simulink model "smallsat_adcs"  (R2025b)
settings: Solver=ode113  StartTime=0.0  StopTime=17403  RelTol=1e-10  AbsTol=1e-10
InitFcn:
  | P = smallsat_params; if ~exist('adcsCase', 'var'), adcsCase = 'tumble'; end; ic = initial_state_case(P, adcsCase); bdot = size_bdot(P); pointing = size_pointing(P);
undefined symbols (not defined in the file or in its folder): DiscIntNeverNeededParam, magnetic_field_eci, quat_to_dcm
libraries: aerolibutil x3, matrix_library x1, simulink x1, sharedutil x1
settings Model: Creator=USER  LastModifiedBy=USER

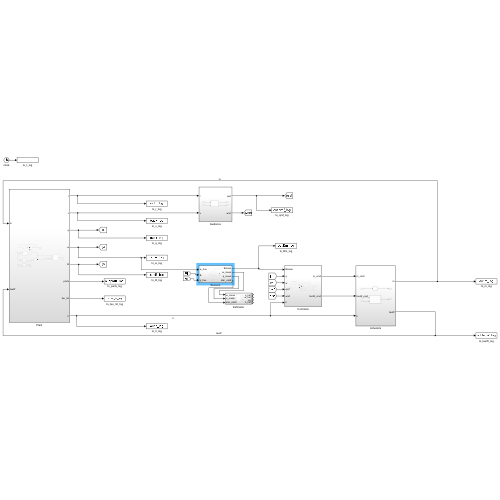
[thumbnail: Simulink's stored preview of the top-level diagram]
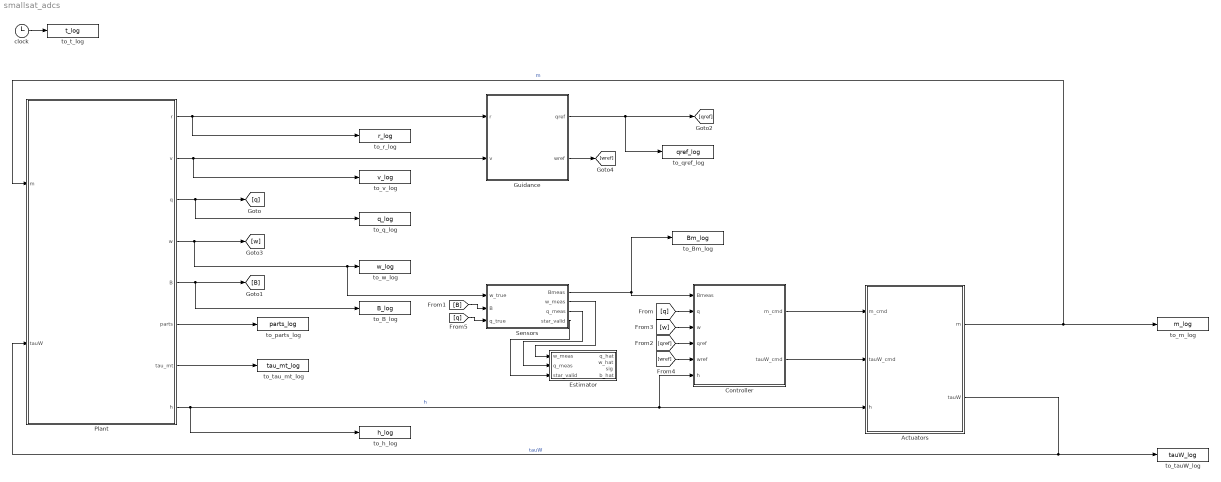
== system smallsat_adcs ==
  Actuators : Subsystem
  Controller : Subsystem
  Estimator : Subsystem
  Guidance : Subsystem
  Plant : Subsystem
  Sensors : Subsystem
  clock : Clock
  to_B_log : ToWorkspace  VariableName=B_log  SampleTime=10
  to_Bm_log : ToWorkspace  VariableName=Bm_log  SampleTime=10
  to_h_log : ToWorkspace  VariableName=h_log  SampleTime=10
  to_m_log : ToWorkspace  VariableName=m_log  SampleTime=10
  to_parts_log : ToWorkspace  VariableName=parts_log  SampleTime=10
  to_q_log : ToWorkspace  VariableName=q_log  SampleTime=10
  to_qref_log : ToWorkspace  VariableName=qref_log  SampleTime=10
  to_r_log : ToWorkspace  VariableName=r_log  SampleTime=10
  to_t_log : ToWorkspace  VariableName=t_log  SampleTime=10
  to_tauW_log : ToWorkspace  VariableName=tauW_log  SampleTime=10
  to_tau_mt_log : ToWorkspace  VariableName=tau_mt_log  SampleTime=10
  to_v_log : ToWorkspace  VariableName=v_log  SampleTime=10
  to_w_log : ToWorkspace  VariableName=w_log  SampleTime=10
  wires:
  Plant/5(B) -> to_B_log/1, [B]
  Plant/1(r) -> Guidance/1(r), to_r_log/1
  Plant/2(v) -> to_v_log/1, Guidance/2(v)
  Sensors/1(Bmeas) -> Controller/1(Bmeas), to_Bm_log/1
  Plant/3(q) -> to_q_log/1, [q]
  Guidance/1(qref) -> to_qref_log/1, [qref]
  Controller/1(m_cmd) -> Actuators/1(m_cmd)
  Controller/2(tauW_cmd) -> Actuators/2(tauW_cmd)
  Plant/8(h) -> to_h_log/1, Actuators/3(h), Controller/6(h)  "h"
  Actuators/1(m) -> to_m_log/1, Plant/1(m)  "m"
  Actuators/2(tauW) -> to_tauW_log/1, Plant/2(tauW)  "tauW"
  clock/1 -> to_t_log/1
  Plant/6(parts) -> to_parts_log/1
  Plant/7(tau_mt) -> to_tau_mt_log/1
  [q] -> Controller/2(q)
  [B] -> Sensors/2(B)
  [qref] -> Controller/4(qref)
  [w] -> Controller/3(w)
  Guidance/2(wref) -> [wref]
  [wref] -> Controller/5(wref)
  Plant/4(w) -> Sensors/1(w_true), to_w_log/1, [w]
  [q] -> Sensors/3(q_true)
  Sensors/2(w_meas) -> Estimator/1(w_meas)
  Sensors/3(q_meas) -> Estimator/2(q_meas)
  Sensors/4(star_valid) -> Estimator/3(star_valid)

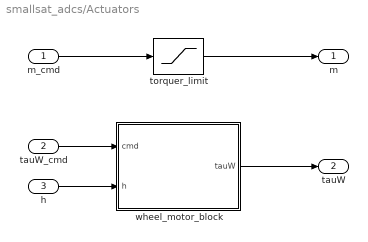
== system smallsat_adcs/Actuators ==
  m_cmd : Inport
  tauW_cmd : Inport  Port=2
  h : Inport  Port=3
  torquer_limit : Saturate  UpperLimit=P.mtqMax  LowerLimit=-P.mtqMax
  wheel_motor_block : MATLAB Function  TreatAsAtomicUnit=on
  m : Outport
  tauW : Outport  Port=2
  wires:
  m_cmd/1 -> torquer_limit/1
  torquer_limit/1 -> m/1
  tauW_cmd/1 -> wheel_motor_block/1(cmd)
  h/1 -> wheel_motor_block/2(h)
  wheel_motor_block/1(tauW) -> tauW/1

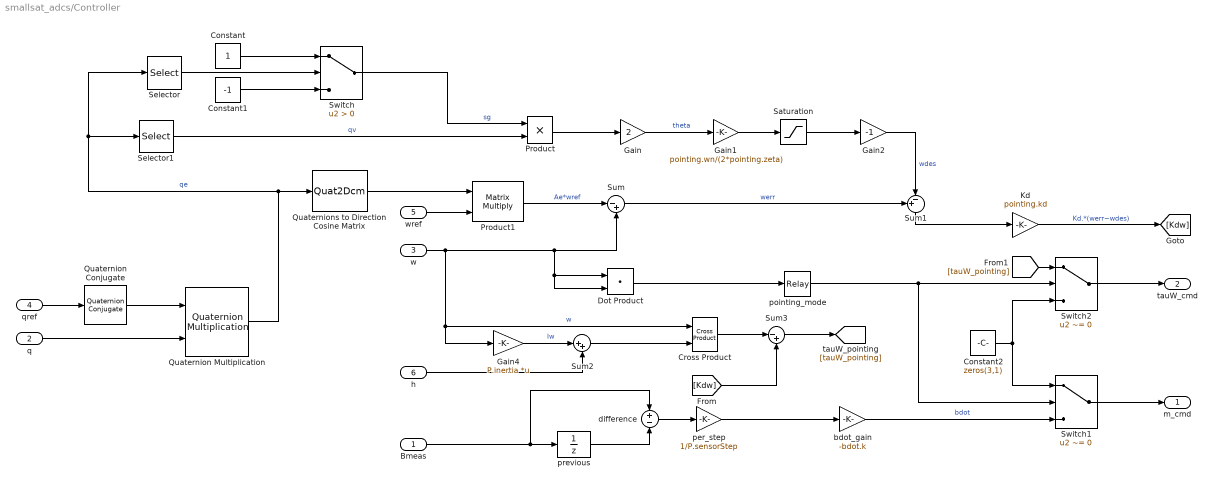
== system smallsat_adcs/Controller ==
  Bmeas : Inport
  q : Inport  Port=2
  w : Inport  Port=3
  qref : Inport  Port=4
  wref : Inport  Port=5
  h : Inport  Port=6
  Constant : Constant
  Constant1 : Constant  Value=-1
  Constant2 : Constant  Value=zeros(3,1)  VectorParams1D=off
  Cross Product : matrix_library/Cross Product
  Dot Product : DotProduct  OutDataTypeStr=Inherit: Inherit via internal rule
  Gain : Gain  Gain=2
  Gain1 : Gain  Gain=pointing.wn/(2*pointing.zeta)
  Gain2 : Gain  Gain=-1
  Gain4 : Gain  Gain=P.inertia  Multiplication=Matrix(K*u)
  Kd : Gain  Gain=pointing.kd
  Product : Product
  Product1 : Product  Multiplication=Matrix(*)
  Quaternion Conjugate : aerolibutil/Quaternion Conjugate
  Quaternion Multiplication : aerolibutil/Quaternion Multiplication
  Quaternions to Direction Cosine Matrix : Quat2Dcm
  Saturation : Saturate  UpperLimit=pointing.wSlew  LowerLimit=-pointing.wSlew
  Selector : Selector  InputPortWidth=4  IndexOptions=Index vector (dialog)  Indices=1  OutputSizes=1
  Selector1 : Selector  InputPortWidth=4  IndexOptions=Index vector (dialog)  Indices=[2 3 4]  OutputSizes=1
  Sum : Sum  Inputs=|-+
  Sum1 : Sum  Inputs=+-|
  Sum2 : Sum  Inputs=|++
  Sum3 : Sum  Inputs=|-+
  Switch : Switch  Criteria=u2 > Threshold  SaturateOnIntegerOverflow=off  InputSameDT=off
  Switch1 : Switch  Criteria=u2 ~= 0  SaturateOnIntegerOverflow=off  InputSameDT=off
  Switch2 : Switch  Criteria=u2 ~= 0  SaturateOnIntegerOverflow=off  InputSameDT=off
  bdot_gain : Gain  Gain=-bdot.k
  difference : Sum  Inputs=+-
  per_step : Gain  Gain=1/P.sensorStep
  pointing_mode : Relay  OnSwitchValue=P.detumbleExit^2  OffSwitchValue=P.detumbleTarget^2  OnOutputValue=0  OffOutputValue=1
  previous : UnitDelay  InitialCondition=quat_to_dcm(ic.q)*magnetic_field_eci(ic.r, 0, P)  SampleTime=P.sensorStep  HasFrameUpgradeWarning=on
  m_cmd : Outport
  tauW_cmd : Outport  Port=2
  wires:
  w/1 -> Cross Product/1, Gain4/1, Sum/2, Dot Product/2, Dot Product/1  "w"
  wref/1 -> Product1/2
  Bmeas/1 -> difference/1, previous/1
  previous/1 -> difference/2
  difference/1 -> per_step/1
  per_step/1 -> bdot_gain/1
  bdot_gain/1 -> Switch1/3  "bdot"
  Switch2/1 -> tauW_cmd/1
  qref/1 -> Quaternion Conjugate/1
  Quaternion Conjugate/1 -> Quaternion Multiplication/1
  q/1 -> Quaternion Multiplication/2
  Quaternion Multiplication/1 -> Quaternions to Direction Cosine Matrix/1, Selector/1, Selector1/1  "qe"
  Constant/1 -> Switch/1
  Selector/1 -> Switch/2
  Constant1/1 -> Switch/3
  Switch/1 -> Product/1  "sg"
  Selector1/1 -> Product/2  "qv"
  Product/1 -> Gain/1
  Gain/1 -> Gain1/1  "theta"
  Gain1/1 -> Saturation/1
  Saturation/1 -> Gain2/1
  Gain2/1 -> Sum1/2  "wdes"
  Quaternions to Direction Cosine Matrix/1 -> Product1/1
  Product1/1 -> Sum/1  "Ae*wref"
  Sum/1 -> Sum1/1  "werr"
  Sum1/1 -> Kd/1
  Kd/1 -> [Kdw]  "Kd.*(werr−wdes)"
  Dot Product/1 -> pointing_mode/1
  Constant2/1 -> Switch2/3, Switch1/1
  pointing_mode/1 -> Switch2/2, Switch1/2
  Switch1/1 -> m_cmd/1
  Gain4/1 -> Sum2/1  "Iw"
  h/1 -> Sum2/2
  Sum2/1 -> Cross Product/2
  Cross Product/1 -> Sum3/1
  [Kdw] -> Sum3/2
  Sum3/1 -> [tauW_pointing]
  [tauW_pointing] -> Switch2/1

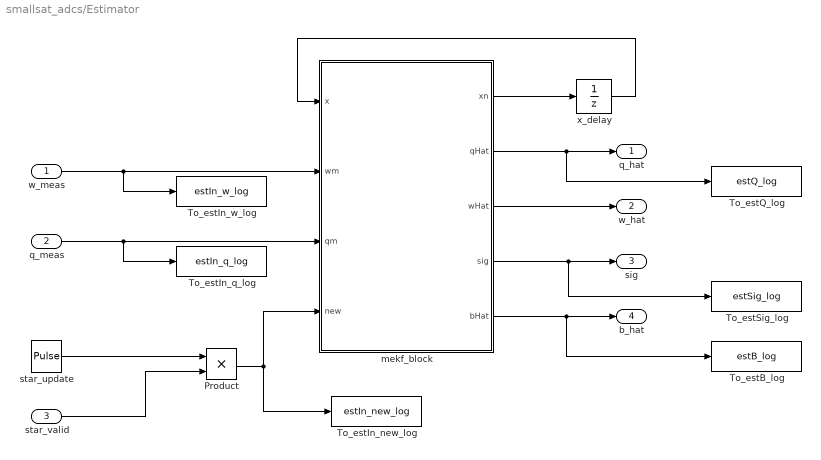
== system smallsat_adcs/Estimator ==
  w_meas : Inport
  q_meas : Inport  Port=2
  star_valid : Inport  Port=3
  Product : Product
  To_estB_log : ToWorkspace  VariableName=estB_log  SampleTime=-1
  To_estIn_new_log : ToWorkspace  VariableName=estIn_new_log  SampleTime=-1
  To_estIn_q_log : ToWorkspace  VariableName=estIn_q_log  SampleTime=P.gyroStep
  To_estIn_w_log : ToWorkspace  VariableName=estIn_w_log  SampleTime=-1
  To_estQ_log : ToWorkspace  VariableName=estQ_log  SampleTime=-1
  To_estSig_log : ToWorkspace  VariableName=estSig_log  SampleTime=-1
  mekf_block : MATLAB Function  TreatAsAtomicUnit=on
  "star_update " : DiscretePulseGenerator  Period=round(P.starStep/P.gyroStep)  SampleTime=P.gyroStep
  x_delay : UnitDelay  InitialCondition=zeros(43,1)  SampleTime=P.gyroStep  HasFrameUpgradeWarning=on
  q_hat : Outport
  w_hat : Outport  Port=2
  sig : Outport  Port=3
  b_hat : Outport  Port=4
  wires:
  "star_update "/1 -> Product/1
  mekf_block/1(xn) -> x_delay/1
  x_delay/1 -> mekf_block/1(x)
  mekf_block/2(qHat) -> q_hat/1, To_estQ_log/1
  mekf_block/3(wHat) -> w_hat/1
  mekf_block/4(sig) -> To_estSig_log/1, sig/1
  mekf_block/5(bHat) -> To_estB_log/1, b_hat/1
  w_meas/1 -> To_estIn_w_log/1, mekf_block/2(wm)
  q_meas/1 -> To_estIn_q_log/1, mekf_block/3(qm)
  star_valid/1 -> Product/2
  Product/1 -> mekf_block/4(new), To_estIn_new_log/1

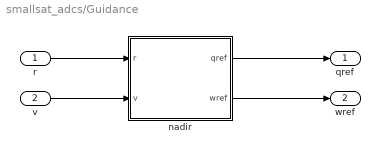
== system smallsat_adcs/Guidance ==
  r : Inport
  v : Inport  Port=2
  nadir : MATLAB Function  TreatAsAtomicUnit=on
  qref : Outport
  wref : Outport  Port=2
  wires:
  r/1 -> nadir/1(r)
  v/1 -> nadir/2(v)
  nadir/1(qref) -> qref/1
  nadir/2(wref) -> wref/1

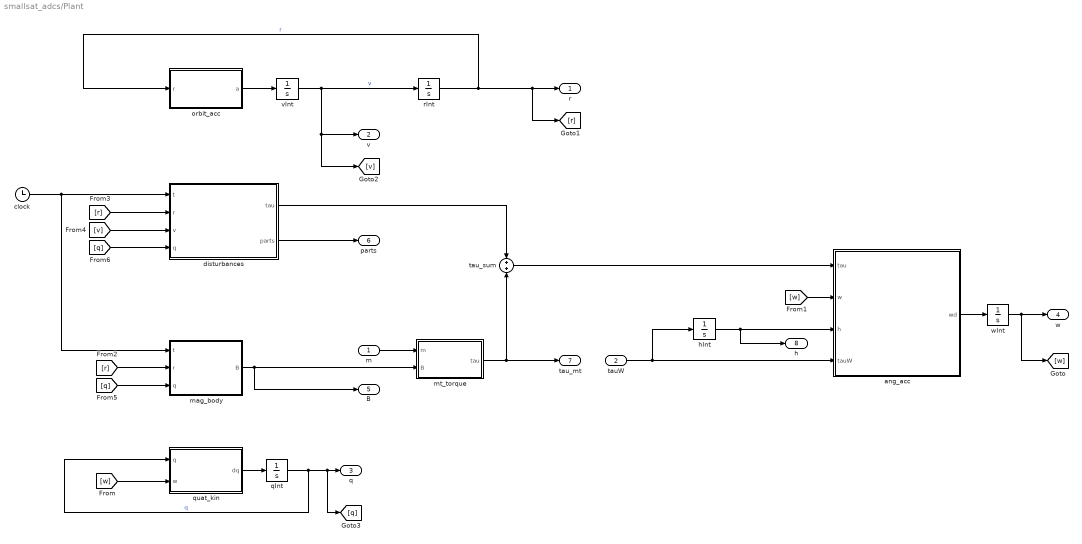
== system smallsat_adcs/Plant ==
  m : Inport
  tauW : Inport  Port=2
  ang_acc : MATLAB Function  TreatAsAtomicUnit=on
  clock : Clock
  disturbances : MATLAB Function  TreatAsAtomicUnit=on
  hInt : Integrator  InitialCondition=ic.h
  mag_body : MATLAB Function  TreatAsAtomicUnit=on
  mt_torque : MATLAB Function  TreatAsAtomicUnit=on
  orbit_acc : MATLAB Function  TreatAsAtomicUnit=on
  qInt : Integrator  InitialCondition=ic.q
  quat_kin : MATLAB Function  TreatAsAtomicUnit=on
  rInt : Integrator  InitialCondition=ic.r
  tau_sum : Sum
  vInt : Integrator  InitialCondition=ic.v
  wInt : Integrator  InitialCondition=ic.w
  r : Outport
  v : Outport  Port=2
  q : Outport  Port=3
  w : Outport  Port=4
  B : Outport  Port=5
  parts : Outport  Port=6
  tau_mt : Outport  Port=7
  h : Outport  Port=8
  wires:
  orbit_acc/1(a) -> vInt/1
  vInt/1 -> rInt/1, [v], v/1  "v"
  clock/1 -> disturbances/1(t), mag_body/1(t)
  qInt/1 -> quat_kin/1(q), [q], q/1  "q"
  m/1 -> mt_torque/1(m)
  mag_body/1(B) -> B/1, mt_torque/2(B)
  disturbances/1(tau) -> tau_sum/1
  mt_torque/1(tau) -> tau_mt/1, tau_sum/2
  tau_sum/1 -> ang_acc/1(tau)
  wInt/1 -> [w], w/1
  hInt/1 -> h/1, ang_acc/3(h)
  tauW/1 -> hInt/1, ang_acc/4(tauW)
  ang_acc/1(wd) -> wInt/1
  quat_kin/1(dq) -> qInt/1
  disturbances/2(parts) -> parts/1
  [w] -> quat_kin/2(w)
  [w] -> ang_acc/2(w)
  [r] -> mag_body/2(r)
  [r] -> disturbances/2(r)
  rInt/1 -> [r], r/1, orbit_acc/1(r)  "r"
  [v] -> disturbances/3(v)
  [q] -> mag_body/3(q)
  [q] -> disturbances/4(q)

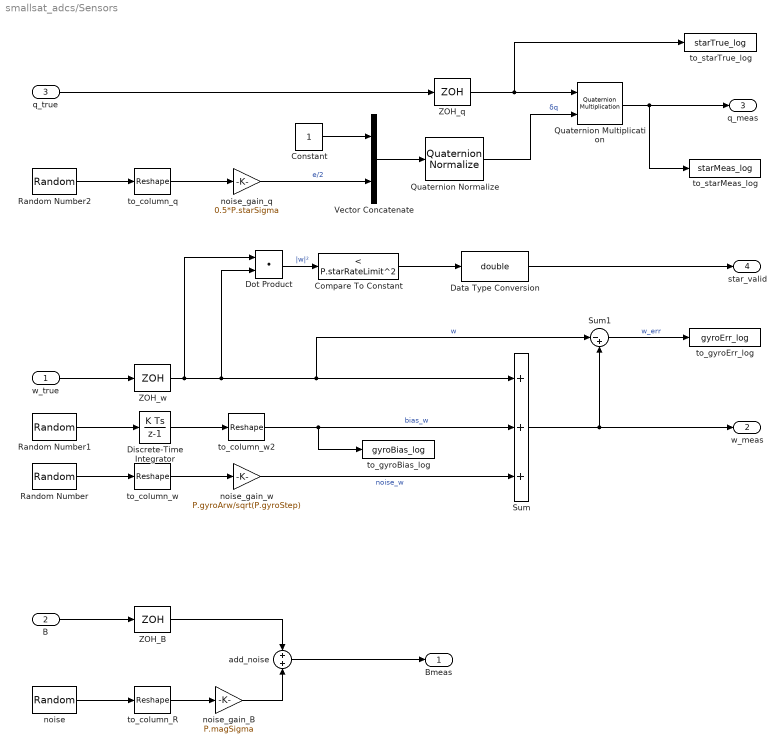
== system smallsat_adcs/Sensors ==
  w_true : Inport
  B : Inport  Port=2
  q_true : Inport  Port=3
  Compare To Constant : simulink/Logic and Bit Operations/Compare To Constant  relop=<  const=P.starRateLimit^2  OutDataTypeStr=boolean
  Constant : Constant
  Data Type Conversion : DataTypeConversion  OutDataTypeStr=double  SaturateOnIntegerOverflow=off  RndMeth=Floor
  Discrete-Time Integrator : DiscreteIntegrator  gainval=P.gyroRrw/sqrt(P.gyroStep)  InitialCondition=P.gyroBias0  SampleTime=P.gyroStep  ICPrevOutput=DiscIntNeverNeededParam  ICPrevScaledInput=DiscIntNeverNeededParam
  Dot Product : DotProduct  OutDataTypeStr=Inherit: Inherit via internal rule
  Quaternion Multiplication : aerolibutil/Quaternion Multiplication
  Quaternion Normalize : sharedutil/Quaternion Normalize  aMode=aMode
  Random Number : RandomNumber  Seed=[41 42 43]  SampleTime=P.gyroStep
  Random Number1 : RandomNumber  Seed=[51 52 53]  SampleTime=P.gyroStep
  Random Number2 : RandomNumber  Seed=[61 62 63]  SampleTime=P.starStep
  Sum : Sum  Inputs=+++
  Sum1 : Sum  Inputs=|-+
  Vector Concatenate : Concatenate
  ZOH_B : ZeroOrderHold  SampleTime=P.sensorStep
  ZOH_q : ZeroOrderHold  SampleTime=P.starStep
  ZOH_w : ZeroOrderHold  SampleTime=P.gyroStep
  add_noise : Sum
  noise : RandomNumber  Seed=[11 22 33]  SampleTime=P.sensorStep
  noise_gain_B : Gain  Gain=P.magSigma
  noise_gain_q : Gain  Gain=0.5*P.starSigma
  noise_gain_w : Gain  Gain=P.gyroArw/sqrt(P.gyroStep)
  to_column_R : Reshape  OutputDimensionality=Customize  OutputDimensions=[3 1]
  to_column_q : Reshape  OutputDimensionality=Customize  OutputDimensions=[3 1]
  to_column_w : Reshape  OutputDimensionality=Customize  OutputDimensions=[3 1]
  to_column_w2 : Reshape  OutputDimensionality=Customize  OutputDimensions=[3 1]
  to_gyroBias_log : ToWorkspace  VariableName=gyroBias_log  SampleTime=-1
  to_gyroErr_log : ToWorkspace  VariableName=gyroErr_log  SampleTime=-1
  to_starMeas_log : ToWorkspace  VariableName=starMeas_log  SampleTime=-1
  to_starTrue_log : ToWorkspace  VariableName=starTrue_log  SampleTime=-1
  Bmeas : Outport
  w_meas : Outport  Port=2
  q_meas : Outport  Port=3
  star_valid : Outport  Port=4
  wires:
  B/1 -> ZOH_B/1
  ZOH_B/1 -> add_noise/1
  noise/1 -> to_column_R/1
  to_column_R/1 -> noise_gain_B/1
  noise_gain_B/1 -> add_noise/2
  add_noise/1 -> Bmeas/1
  w_true/1 -> ZOH_w/1
  Random Number/1 -> to_column_w/1
  to_column_w/1 -> noise_gain_w/1
  Random Number1/1 -> Discrete-Time Integrator/1
  Discrete-Time Integrator/1 -> to_column_w2/1
  noise_gain_w/1 -> Sum/3  "noise_w"
  ZOH_w/1 -> Dot Product/1, Dot Product/2, Sum1/1, Sum/1  "w"
  Sum/1 -> w_meas/1, Sum1/2
  Sum1/1 -> to_gyroErr_log/1  "w_err"
  q_true/1 -> ZOH_q/1
  ZOH_q/1 -> to_starTrue_log/1, Quaternion Multiplication/1
  to_column_w2/1 -> to_gyroBias_log/1, Sum/2  "bias_w"
  Random Number2/1 -> to_column_q/1
  to_column_q/1 -> noise_gain_q/1
  noise_gain_q/1 -> Vector Concatenate/2  "e/2"
  Constant/1 -> Vector Concatenate/1
  Vector Concatenate/1 -> Quaternion Normalize/1
  Quaternion Normalize/1 -> Quaternion Multiplication/2  "δq"
  Quaternion Multiplication/1 -> to_starMeas_log/1, q_meas/1
  Dot Product/1 -> Compare To Constant/1  "|w|²"
  Data Type Conversion/1 -> star_valid/1
  Compare To Constant/1 -> Data Type Conversion/1

== matlab function smallsat_adcs/Plant/disturbances ==
  data: t input; tau output; r input; v input; q input; parts output; P parameter
function [tau, parts] = disturbances(t, r, v, q, P)

[tau, parts] = disturbance_block(t, r, v, q, P);
end

== matlab function smallsat_adcs/Plant/orbit_acc ==
  data: r input; a output; P parameter
function a = orbit_acc(r, P)

a = j2_accel(r, P);
end

== matlab function smallsat_adcs/Plant/mag_body ==
  data: t input; B output; r input; q input; P parameter
function B = mag_body(t, r, q, P)

B = quat_to_dcm(q)*magnetic_field_eci(r, t, P);
end

== matlab function smallsat_adcs/Plant/mt_torque ==
  data: m input; tau output; B input
function tau = mt_torque(m, B)

tau = cross(m, B);
end

== matlab function smallsat_adcs/Plant/ang_acc ==
  data: tau input; wd output; w input; h input; tauW input; P parameter
function wd = ang_acc(tau, w, h, tauW, P)

wd = angular_accel(w, h, tau, tauW, P.inertia);
end

== matlab function smallsat_adcs/Plant/quat_kin ==
  data: q input; dq output; w input
function dq = quat_kin(q, w)

dq = quat_rate(q, w);
end

== matlab function smallsat_adcs/Guidance/nadir ==
  data: r input; qref output; v input; wref output
function [qref, wref] = nadir(r, v)

[qref, wref] = nadir_reference(r, v);
end

== matlab function smallsat_adcs/Actuators/wheel_motor_block ==
  data: cmd input; tauW output; h input; P parameter
function tauW = wheel_motor_block(cmd, h, P)

tauW = wheel_motor(cmd, h, P);
end

== matlab function smallsat_adcs/Estimator/mekf_block ==
  data: x input; xn output; wm input; qm input; new input; qHat output; wHat output; sig output; bHat output; P parameter
function [xn, qHat, wHat, sig, bHat] = mekf_block(x, wm, qm, new, P)

xn = mekf_step(x, wm, qm, new, P);
[qHat, wHat, sig, bHat] = mekf_outputs(xn, wm, qm);
end
